simulink model "rotacional_sim"  (R2022b)
settings: Solver=VariableStepAuto  StartTime=0.0  StopTime=10.0  FixedStep=0.01  RelTol=1e-3
values from neighbouring files (symbols this model uses):
  b1 = 1    [rotacional.m]
  b2 = 1    [rotacional.m]
  j1 = 1    [rotacional.m]
  j2 = 1    [rotacional.m]
  k = 0.1    [rotacional.m]
settings Model: Creator=Fran  LastModifiedBy=Fran

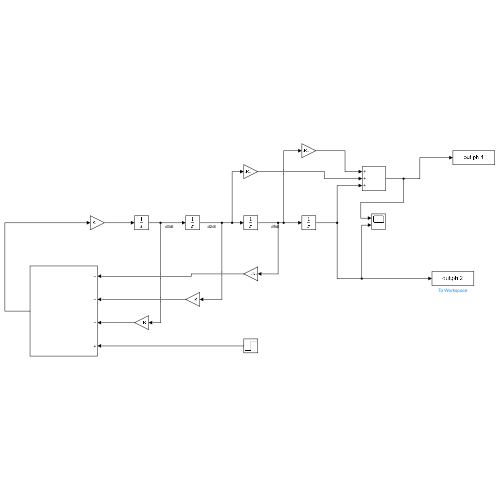
[thumbnail: Simulink's stored preview of the top-level diagram]
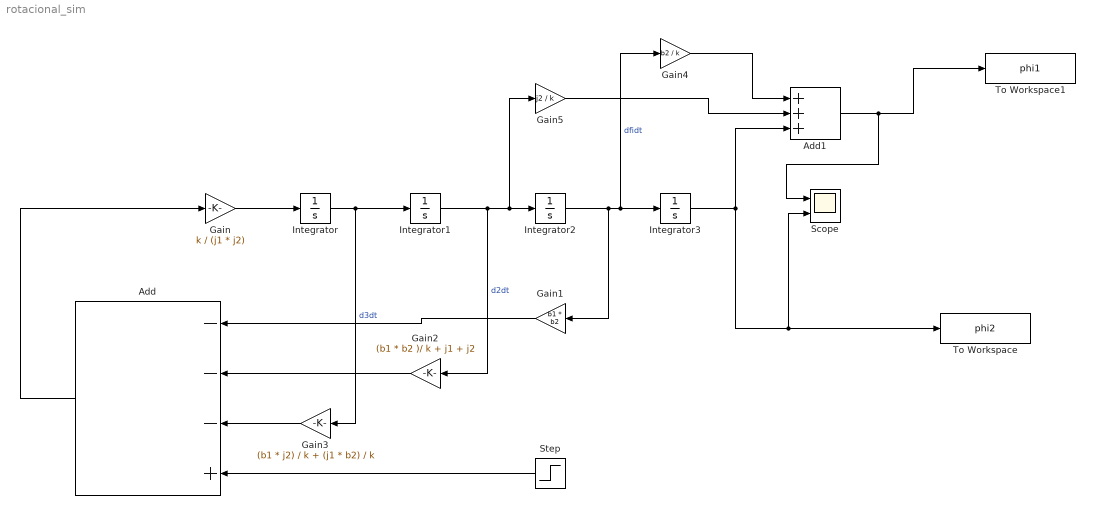
== system rotacional_sim ==
  Add : Sum  Inputs=---+
  Add1 : Sum  Inputs=+++
  Gain : Gain  Gain=k / (j1 * j2)
  Gain1 : Gain  Gain=b1 * b2
  Gain2 : Gain  Gain=(b1 * b2 )/ k + j1 + j2
  Gain3 : Gain  Gain=(b1 * j2) / k + (j1 * b2) / k
  Gain4 : Gain  Gain=b2 / k
  Gain5 : Gain  Gain=j2 / k
  Integrator{,1..3} (4 alike) : Integrator
  Scope : Scope  NumInputPorts=2
  Step : Step  SampleTime=0
  To Workspace : ToWorkspace  VariableName=phi2  SampleTime=-1
  To Workspace1 : ToWorkspace  VariableName=phi1  SampleTime=-1
  wires:
  Integrator/1 -> Gain3/1, Integrator1/1  "d3dt"
  Integrator1/1 -> Gain5/1, Integrator2/1, Gain2/1  "d2dt"
  Integrator2/1 -> Gain1/1, Gain4/1, Integrator3/1  "dfidt"
  Gain/1 -> Integrator/1
  Gain1/1 -> Add/1
  Gain2/1 -> Add/2
  Gain3/1 -> Add/3
  Step/1 -> Add/4
  Add/1 -> Gain/1
  Integrator3/1 -> Add1/3, Scope/2, To Workspace/1
  Gain5/1 -> Add1/2
  Gain4/1 -> Add1/1
  Add1/1 -> Scope/1, To Workspace1/1
